simulink model "main"  (R2020b)
settings: Solver=ode14x  StartTime=0.0  StopTime=300  FixedStep=ContIntTime  RelTol=1e-3
undefined symbols (not defined in the file): EnumPistSt
libraries: autolibshared x1, simulink x1
settings Model: DataDictionary=main.sldd  NumberOfSteps=10  Creator=Dmitry  LastModifiedBy=Dmitry

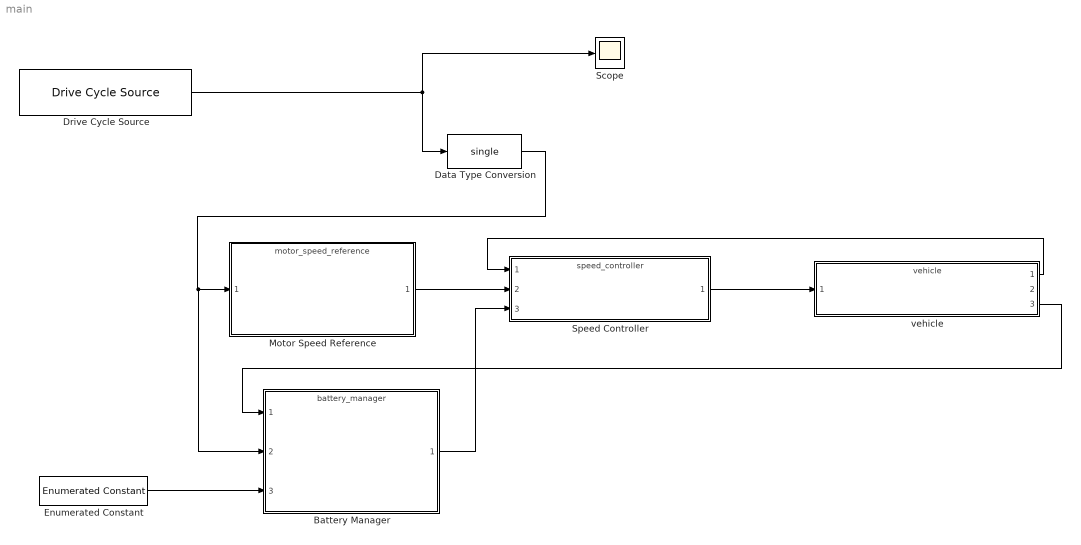
== system main ==
  Battery Manager : ModelReference  ModelNameDialog=battery_manager.slx  SimulationMode=Normal  ModelReferenceVersion=1.61
  Data Type Conversion : DataTypeConversion  OutDataTypeStr=single
  Drive Cycle Source : autolibshared/Drive Cycle Source  cycleVar=FTP75  fileVar=cycleFTP75.mat  tfinal="2474  seconds"  cycleRepeat=off  outAccPort=off  outGearPort=off  gearList=No gear data  t_wot1=5  xdot_woto=0  xdot_wot1=30  t_wot2=20  xdot_wot2=0  t_wotend=30  srcUnit=m/s  outUnit=km/h  srcAccUnit=m/s/s  outAccUnit=m/s^2  dt=0  aMode=1  faultOption=off  velBnd=2  velBndUnit=mph  inUnit=m/s  timeBnd=1  failOption=off  stopSim=off  maxFaultCnt=10  maxFaultTime=2  maxTotFaultTime=15  traceOption=off  dtTrace=1  traceWindow=10  lastDCname=FTP75 Velocity  lastOutUnit=mph  lastDT=0  lastTB=1  lastSB=2  forceCalcBound=off
      settings: SourceProductBaseCode=PW,MT,UV,VE,VP
  Enumerated Constant : simulink/Sources/Enumerated Constant  OutDataTypeStr=Enum: EnumPistSt  Value=EnumPistSt.NA  SampleTime=inf
  Motor Speed Reference : ModelReference  ModelNameDialog=motor_speed_reference.slx  SimulationMode=Normal  ModelReferenceVersion=1.12
  Scope : Scope
  Speed Controller : ModelReference  ModelNameDialog=speed_controller.slx  SimulationMode=Normal  ModelReferenceVersion=1.27
  vehicle : ModelReference  ModelNameDialog=vehicle.slx  SimulationMode=Normal  ModelReferenceVersion=1.44
  wires:
  Speed Controller/1 -> vehicle/1
  Data Type Conversion/1 -> Battery Manager/2, Motor Speed Reference/1
  Motor Speed Reference/1 -> Speed Controller/2
  Drive Cycle Source/1 -> Data Type Conversion/1, Scope/1
  vehicle/1 -> Speed Controller/1
  vehicle/3 -> Battery Manager/1
  Enumerated Constant/1 -> Battery Manager/3
  Battery Manager/1 -> Speed Controller/3
